simulink model "SBC_adv"  (R2023a)
settings: Solver=VariableStepAuto  StartTime=0  StopTime=10  FixedStep=0.002  RelTol=1e-3  AbsTol=1e-6
InitFcn:
  | global t
  | t = 0;
libraries: Solver_SF x1
settings Model: ExtModeTrigMode=oneshot  Creator=ywata  LastModifiedBy=USER
settings SolverCC: AutoScaleAbsTol=off  AlgebraicLoopSolver=TrustRegion
settings DataIOCC: SaveFormat=Array  SignalLoggingSaveFormat=ModelDataLogs  ReturnWorkspaceOutputs=off  SignalLoggingName=sigsOut
settings OptimizationCC: BlockReduction=off  BooleanDataType=off  ExpressionDepthLimit=2147483647  LifeSpan=inf
settings DebuggingCC: SaveWithParameterizedLinksMsg=none  UnderspecifiedInitializationDetection=Classic  MergeDetectMultiDrivingBlocksExec=none  SignalResolutionControl=TryResolveAllWithWarning  MultiTaskDSMMsg=warning  MultiTaskCondExecSysMsg=none  FcnCallInpInsideContextMsg=warning  UnconnectedInputMsg=warning  UnconnectedOutputMsg=warning  UnconnectedLineMsg=warning  StateNameClashWarn=warning  SFUnexpectedBacktrackingDiag=warning  SFNoUnconditionalDefaultTransitionDiag=warning  SFExecutionAtInitializationDiag=none  ArithmeticOperatorsInVariantConditions=warning
settings HardwareCC: ProdBitPerPointer=32  ProdBitPerSizeT=32  ProdBitPerPtrDiffT=32  ProdLargestAtomicFloat=None  ProdIntDivRoundTo=Undefined  ProdEndianess=Unspecified  ProdWordSize=32  ProdHWDeviceType=32-bit Generic  TargetUnknown=on
settings ModelReferenceCC: PropagateSignalLabelsOutOfModel=off
settings SFSimCC: SimUseLocalCustomCode=off  CustomCodeUndefinedFunction=UseInterfaceOnly
settings RTWCC: TemplateMakefile=grt_vc.tmf  RTWUseLocalCustomCode=off
settings CodeAppCC: StateflowObjectComments=on
settings GRTTargetCC: TargetFcnLib=ansi_tfl_tmw.mat  TargetLangStandard=C89/C90 (ANSI)  CombineOutputUpdateFcns=off  GRTInterface=on
settings ConfigComp: CovMetricSettings=dw  CovSaveCumulativeToWorkspaceVar=on  CovSaveSingleToWorkspaceVar=on  CovExternalEMLEnable=off

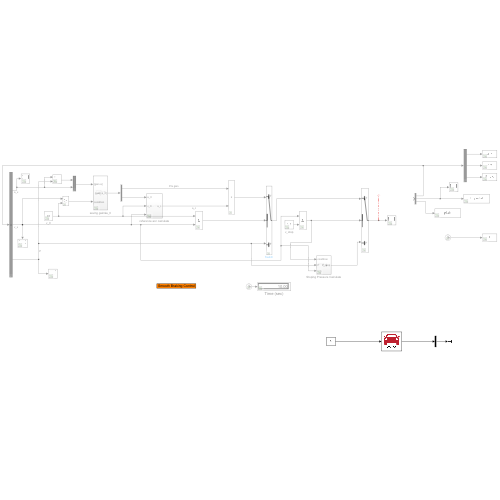
[thumbnail: Simulink's stored preview of the top-level diagram]
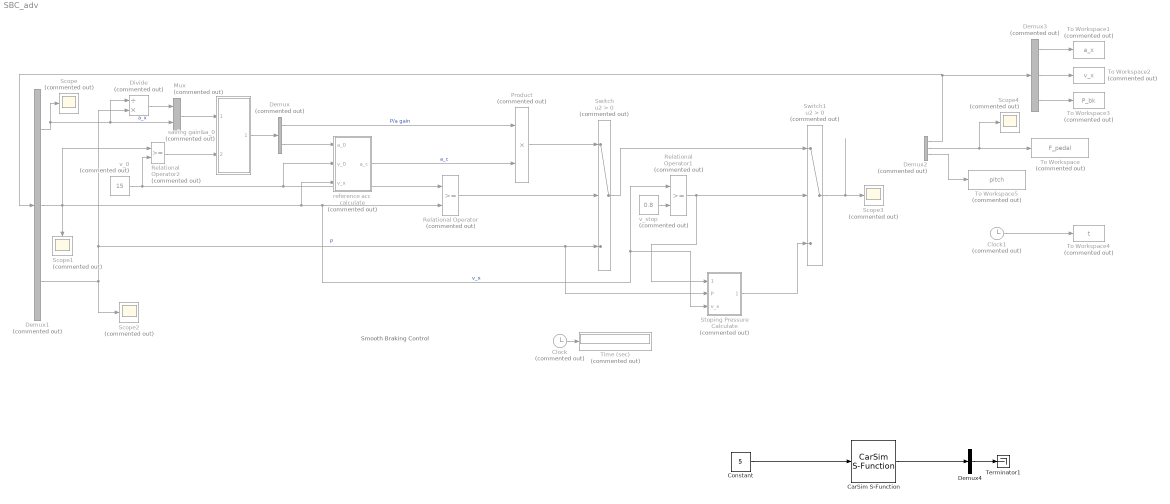
== system SBC_adv ==
  note: Smooth Braking Control
  CarSim S-Function : Solver_SF/CarSim S-Function  Priority=1  SIMFILE=simfile.sim  Run_RTs=off  vs_state_ind=Run  StopMode_ind=Vehicle Model
  Clock : Clock  Commented=on
  Clock1 : Clock  Commented=on
  Constant : Constant  Value=5
  Demux : Demux  Commented=on  Outputs=2
  Demux1 : Demux  Commented=on  Outputs=3
      settings: DisplayOption=none
  Demux2 : Demux  Commented=on  Outputs=[3 1 1]
  Demux3 : Demux  Commented=on  Outputs=3
  Demux4 : Demux  Outputs=[5]
  Divide : Product  Commented=on  Inputs=/*
  Mux : Mux  Commented=on  Inputs=2
  Product : Product  Commented=on
  Relational Operator : RelationalOperator  Commented=on  OutDataTypeStr=boolean  RndMeth=Simplest  InputSameDT=off
  Relational Operator1 : RelationalOperator  Commented=on  OutDataTypeStr=boolean  RndMeth=Simplest  InputSameDT=off
  Relational Operator2 : RelationalOperator  Commented=on  OutDataTypeStr=boolean  RndMeth=Simplest  InputSameDT=off
  Scope{,1..4} (5 alike) : Scope  Commented=on
  Stoping Pressure Calculate : Subsystem  Commented=on
  Switch : Switch  Commented=on  Criteria=u2 > Threshold  SaturateOnIntegerOverflow=off  InputSameDT=off
  Switch1 : Switch  Commented=on  Criteria=u2 > Threshold  SaturateOnIntegerOverflow=off  InputSameDT=off
  Terminator1 : Terminator
  Time (sec) : Display  Commented=on
      settings: Format=bank  Decimation=100
  To Workspace : ToWorkspace  Commented=on  VariableName=F_pedal  SaveFormat=Timeseries  SampleTime=-1
  To Workspace1 : ToWorkspace  Commented=on  VariableName=a_x  SaveFormat=Timeseries  SampleTime=-1
  To Workspace2 : ToWorkspace  Commented=on  VariableName=v_x  SaveFormat=Timeseries  SampleTime=-1
  To Workspace3 : ToWorkspace  Commented=on  VariableName=P_bk  SaveFormat=Timeseries  SampleTime=-1
  To Workspace4 : ToWorkspace  Commented=on  VariableName=t  SaveFormat=Timeseries  SampleTime=-1
  To Workspace5 : ToWorkspace  Commented=on  VariableName=pitch  SaveFormat=Timeseries  SampleTime=-1
  reference acc calculate : Subsystem  Commented=on
  saving gain&a_0 : Subsystem  Commented=on
  v_0 : Constant  Commented=on  Value=15
  v_stop : Constant  Commented=on  Value=0.8
  wires:
  Clock/1 -> Time (sec)/1
  Demux1/3 -> Scope2/1, Divide/2, Stoping Pressure Calculate/2(P), Switch/3  "P"
  Demux1/1 -> Scope/1, Divide/1, Mux/2  "a_x"
  Demux1/2 -> reference acc calculate/3(v_x), Stoping Pressure Calculate/3(v_x), Relational Operator1/1, Relational Operator/2, Scope1/1, Relational Operator2/1  "v_x"
  v_0/1 -> Relational Operator2/2, reference acc calculate/2(v_0), Relational Operator/1
  reference acc calculate/1(a_c) -> Product/2  "a_c"
  Relational Operator/1 -> Switch/2
  Switch/1 -> Switch1/1
  Relational Operator1/1 -> Stoping Pressure Calculate/1(condition), Switch1/2
  v_stop/1 -> Relational Operator1/2
  Divide/1 -> Mux/1
  Demux/2 -> reference acc calculate/1(a_0)
  Product/1 -> Switch/1
  Demux/1 -> Product/1  "P/a gain"
  Switch1/1 -> Scope3/1
  Demux2/1 -> Demux1/1, Demux3/1
  Stoping Pressure Calculate/1(P_stop) -> Switch1/3
  Mux/1 -> saving gain&a_0/1("[gain a]")
  Relational Operator2/1 -> saving gain&a_0/2(condition)
  saving gain&a_0/1("[gain a_0]") -> Demux/1
  CarSim S-Function/1 -> Demux4/1
  Demux2/2 -> Scope4/1, To Workspace/1
  Demux3/1 -> To Workspace1/1
  Demux3/2 -> To Workspace2/1
  Demux3/3 -> To Workspace3/1
  Clock1/1 -> To Workspace4/1
  Constant/1 -> CarSim S-Function/1
  Demux2/3 -> To Workspace5/1
  Demux4/1 -> Terminator1/1

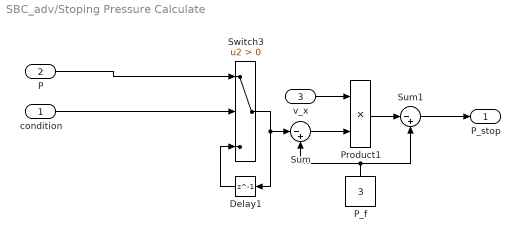
== system SBC_adv/Stoping Pressure Calculate ==
  condition : Inport
  P : Inport  Port=2
  v_x : Inport  Port=3
  Delay1 : Delay  DelayLength=1  InitialCondition=0
  P_f : Constant  Value=3
  Product1 : Product
  Sum : Sum  Inputs=|-+
  Sum1 : Sum  Inputs=|-+
  Switch3 : Switch  Criteria=u2 > Threshold  SaturateOnIntegerOverflow=off  InputSameDT=off
  P_stop : Outport
  wires:
  Product1/1 -> Sum1/1
  Switch3/1 -> Sum/1, Delay1/1
  Delay1/1 -> Switch3/3
  condition/1 -> Switch3/2
  P_f/1 -> Sum/2, Sum1/2
  Sum1/1 -> P_stop/1
  Sum/1 -> Product1/2
  P/1 -> Switch3/1
  v_x/1 -> Product1/1

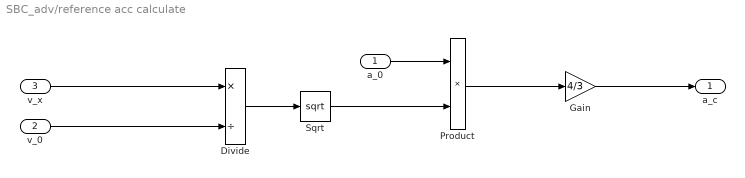
== system SBC_adv/reference acc calculate ==
  a_0 : Inport
  v_0 : Inport  Port=2
  v_x : Inport  Port=3
  Divide : Product  Inputs=*/
  Gain : Gain  Gain=4/3
  Product : Product
  Sqrt : Sqrt
  a_c : Outport
  wires:
  v_x/1 -> Divide/1
  v_0/1 -> Divide/2
  Divide/1 -> Sqrt/1
  Sqrt/1 -> Product/2
  a_0/1 -> Product/1
  Product/1 -> Gain/1
  Gain/1 -> a_c/1

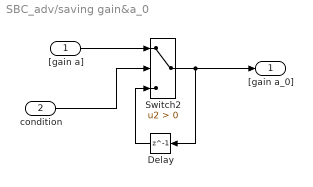
== system SBC_adv/saving gain&a_0 ==
  "[gain a]" : Inport
  condition : Inport  Port=2
  Delay : Delay  DelayLength=1  InitialCondition=0
  Switch2 : Switch  Criteria=u2 > Threshold  SaturateOnIntegerOverflow=off  InputSameDT=off
  "[gain a_0]" : Outport
  wires:
  Switch2/1 -> "[gain a_0]"/1, Delay/1
  Delay/1 -> Switch2/3
  condition/1 -> Switch2/2
  "[gain a]"/1 -> Switch2/1
